simulink model "testtest11"  (Simulink 7.6)
settings: Solver=ode45  StartTime=0.0  StopTime=2000  RelTol=1e-3
values from neighbouring files (symbols this model uses):
  K = [9.375  -6.25; -8.125  8.75]    [PP2013428.mat]
libraries: ADRC x2
settings Model: Creator=Administrator  LastModifiedBy=Administrator
settings DebuggingCC: AlgebraicLoopMsg=none  ArtificialAlgebraicLoopMsg=none  SolverPrmCheckMsg=none  UnknownTsInhSupMsg=none

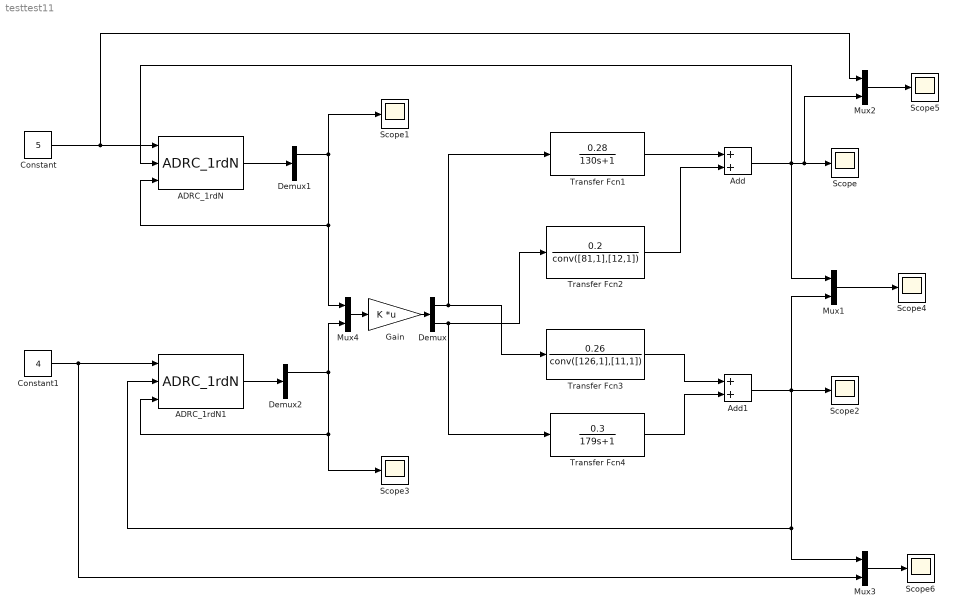
== system testtest11 ==
  ADRC_1rdN : ADRC/ADRC/ADRC_1rd/ADRC_1rdN  SystemSampleTime=-1  RT=500  h=0.1  B01=10  B02=200  r=0.5
  ADRC_1rdN1 : ADRC/ADRC/ADRC_1rd/ADRC_1rdN  SystemSampleTime=-1  RT=500  h=0.1  B01=10  B02=200  r=0.5
  Add : Sum
  Add1 : Sum
  Constant : Constant  Value=5
  Constant1 : Constant  Value=4
  Demux : Demux  Outputs=2
  Demux1 : Demux  Outputs=2
  Demux2 : Demux  Outputs=2
  Gain : Gain  Gain=K  Multiplication=Matrix(K*u)
  Mux{1..4} (4 alike) : Mux  Inputs=2
  Scope{,1..6} (7 alike) : Scope
      Scope settings: TimeRange=1000  YMin=-2e+235  YMax=1.4e+236  DataFormat=Array
      Scope1 settings: YMin=0  YMax=250  DataFormat=Array
      Scope2 settings: YMin=5.25  YMax=10.25  SaveName=ScopeData2  DataFormat=Array
      Scope3 settings: YMin=0  YMax=250  SaveName=ScopeData3  DataFormat=Array
      Scope4 settings: TimeRange=1000  YMin=-2e+235  YMax=1.4e+236  SaveName=ScopeData4  DataFormat=Array
      Scope5 settings: TimeRange=1000  YMin=-2e+235  YMax=1.4e+236  SaveName=ScopeData5  DataFormat=Array
      Scope6 settings: TimeRange=1000  YMin=-2e+235  YMax=1.4e+236  SaveName=ScopeData6  DataFormat=Array
  Transfer Fcn1 : TransferFcn  Numerator=0.28  Denominator=[130 1]
  Transfer Fcn2 : TransferFcn  Numerator=0.2  Denominator=conv([81,1],[12,1])
  Transfer Fcn3 : TransferFcn  Numerator=0.26  Denominator=conv([126,1],[11,1])
  Transfer Fcn4 : TransferFcn  Numerator=0.3  Denominator=[179,1]
  wires:
  Constant/1 -> ADRC_1rdN/1, Mux2/1
  ADRC_1rdN/1 -> Demux1/1
  Mux4/1 -> Gain/1
  Gain/1 -> Demux/1
  Demux/1 -> Transfer Fcn1/1, Transfer Fcn3/1
  Transfer Fcn1/1 -> Add/1
  Transfer Fcn2/1 -> Add/2
  Add/1 -> ADRC_1rdN/2, Mux1/1, Scope/1, Mux2/2
  Transfer Fcn3/1 -> Add1/1
  Transfer Fcn4/1 -> Add1/2
  Add1/1 -> Scope2/1, Mux1/2, ADRC_1rdN1/2, Mux3/1
  Constant1/1 -> ADRC_1rdN1/1, Mux3/2
  Demux1/1 -> Mux4/1, ADRC_1rdN/3, Scope1/1
  ADRC_1rdN1/1 -> Demux2/1
  Demux2/1 -> Mux4/2, ADRC_1rdN1/3, Scope3/1
  Demux/2 -> Transfer Fcn2/1, Transfer Fcn4/1
  Mux1/1 -> Scope4/1
  Mux2/1 -> Scope5/1
  Mux3/1 -> Scope6/1
